simulink model "problem_2c"  (R2018a)
settings: Solver=VariableStepAuto  StartTime=0.0  StopTime=10  MaxStep=1e-3  RelTol=1e-3
values from neighbouring files (symbols this model uses):
  dx0 = 5    [distance_x.m]    (also in grid_search_minimization.m = sqrt(2/m*(Esys-m*g*y0)); minimization.m = sqrt(2/m*(Esys-m*g*y0)); problem_1_script.m; problem_3_script.m = sqrt(2/m*(Esys-m*g*y0)))
  dy0 = 0    [distance_x.m]    (also in grid_search_minimization.m; minimization.m; problem_1_script.m; problem_3_script.m)
  g = 9.81    [distance_x.m]    (also in grid_search_minimization.m; minimization.m; problem_1_script.m; problem_3_script.m)
  ground = 0.00001    (= 1e-05)    [problem_1_script.m]    (also in problem_3_script.m; smm_params.m)
  k = 20000    [distance_x.m]    (also in grid_search_minimization.m = kVec(kIdx); minimization.m; problem_1_script.m = kVec(kIdx); problem_3_script.m)
  l0 = 1    [distance_x.m]    (also in grid_search_minimization.m; minimization.m; problem_1_script.m; problem_3_script.m)
  m = 80    [distance_x.m]    (also in grid_search_minimization.m; minimization.m; problem_1_script.m; problem_3_script.m)
  x0 = 0    [distance_x.m]    (also in grid_search_minimization.m; minimization.m; problem_1_script.m; problem_3_script.m)
  y0 = 1    [distance_x.m]    (also in grid_search_minimization.m = y0Vec(yIdx); minimization.m = y0Vec(yIdx); problem_1_script.m; problem_3_script.m = y0Vec3(yIdx))
undefined symbols (not defined in the file or in its folder): angle_noise
libraries: simulink_extras x1
settings Model: Creator=hgeyer  LastModifiedBy=oliver

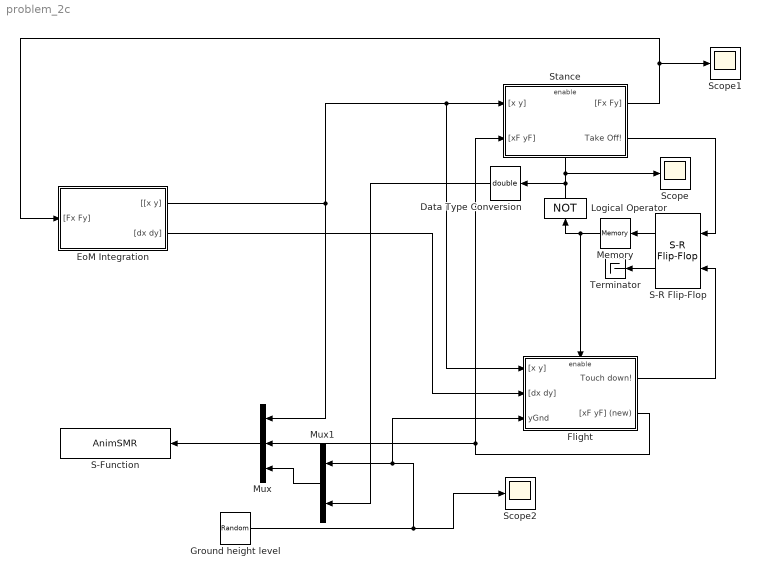
== system problem_2c ==
  " Stance" : Subsystem
  Data Type Conversion : DataTypeConversion  OutDataTypeStr=double
  EoM Integration : Subsystem
  Flight : Subsystem
  Ground height level : UniformRandomNumber  Minimum=-ground  Maximum=ground  SampleTime=0.3
  Logical Operator : Logic  Operator=NOT  AllPortsSameDT=off  OutDataTypeStr=boolean
  Memory : Memory  InitialCondition=1
  Mux : Mux  Inputs=3
  Mux1 : Mux  Inputs=2
  S-Function : S-Function  FunctionName=AnimSMR  Parameters=0.5  SFunctionDeploymentMode=off  EnableBusSupport=off
  S-R Flip-Flop : simulink_extras/Flip Flops/S-R Flip-Flop  initial_condition=1
  Scope : Scope
  Scope1 : Scope
  Scope2 : Scope
  Terminator : Terminator
  wires:
  EoM Integration/1("[[x y]") -> Flight/1("[x y]"), " Stance"/1("[x y]"), Mux/1
  EoM Integration/2("[dx dy]") -> Flight/2("[dx dy]")
  " Stance"/2(Take Off!) -> S-R Flip-Flop/1
  S-R Flip-Flop/1 -> Memory/1
  Logical Operator/1 -> Data Type Conversion/1, " Stance"/Enable, Scope/1
  Memory/1 -> Logical Operator/1, Flight/Enable
  S-R Flip-Flop/2 -> Terminator/1
  Flight/1(Touch down!) -> S-R Flip-Flop/2
  " Stance"/1("[Fx Fy]") -> EoM Integration/1("[Fx Fy]"), Scope1/1
  Flight/2("[xF yF] (new)") -> " Stance"/2("[xF yF]"), Mux/2
  Mux/1 -> S-Function/1
  Mux1/1 -> Mux/3
  Data Type Conversion/1 -> Mux1/2
  Ground height level/1 -> Flight/3(yGnd), Mux1/1, Scope2/1

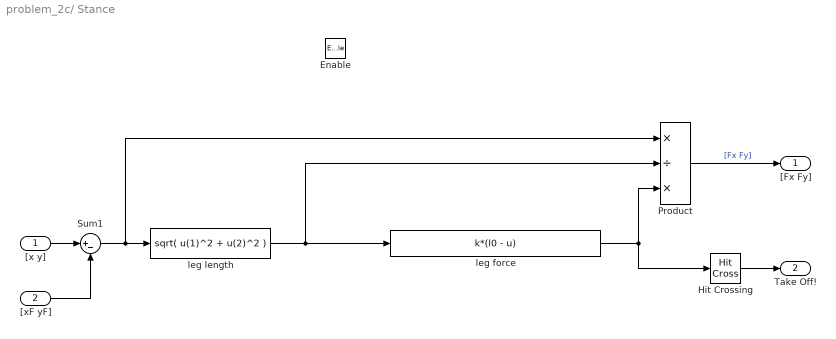
== system problem_2c/ Stance ==
  "[x y]" : Inport
  "[xF yF]" : Inport  Port=2
  Enable : EnablePort
  Hit Crossing : HitCross  HitCrossingDirection=falling
  Product : Product  Inputs=*/*
  Sum1 : Sum  Inputs=|+-
  leg force : Fcn  Expr=k*(l0 - u)
  leg length : Fcn  Expr=sqrt( u(1)^2 + u(2)^2 )
  "[Fx Fy]" : Outport  OutputWhenDisabled=reset  InitialOutput=[0,0]
  Take Off! : Outport  Port=2  OutputWhenDisabled=reset  InitialOutput=0
  wires:
  Product/1 -> "[Fx Fy]"/1  "[Fx Fy]"
  leg length/1 -> leg force/1, Product/2
  Hit Crossing/1 -> Take Off!/1
  "[x y]"/1 -> Sum1/1
  "[xF yF]"/1 -> Sum1/2
  Sum1/1 -> Product/1, leg length/1
  leg force/1 -> Hit Crossing/1, Product/3

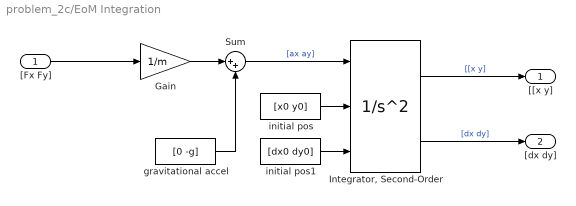
== system problem_2c/EoM Integration ==
  "[Fx Fy]" : Inport
  Gain : Gain  Gain=1/m
  "Integrator, Second-Order" : SecondOrderIntegrator  ICSourceX=external  ICSourceDXDT=external
  Sum : Sum  Inputs=|++
  gravitational accel : Constant  Value=[0 -g]
  initial pos : Constant  Value=[x0 y0]
  initial pos1 : Constant  Value=[dx0 dy0]
  "[[x y]" : Outport
  "[dx dy]" : Outport  Port=2
  wires:
  "[Fx Fy]"/1 -> Gain/1
  initial pos1/1 -> "Integrator, Second-Order"/3
  "Integrator, Second-Order"/2 -> "[dx dy]"/1  "[dx dy]"
  Gain/1 -> Sum/1
  initial pos/1 -> "Integrator, Second-Order"/2
  "Integrator, Second-Order"/1 -> "[[x y]"/1  "[[x y]"
  Sum/1 -> "Integrator, Second-Order"/1  "[ax ay]"
  gravitational accel/1 -> Sum/2

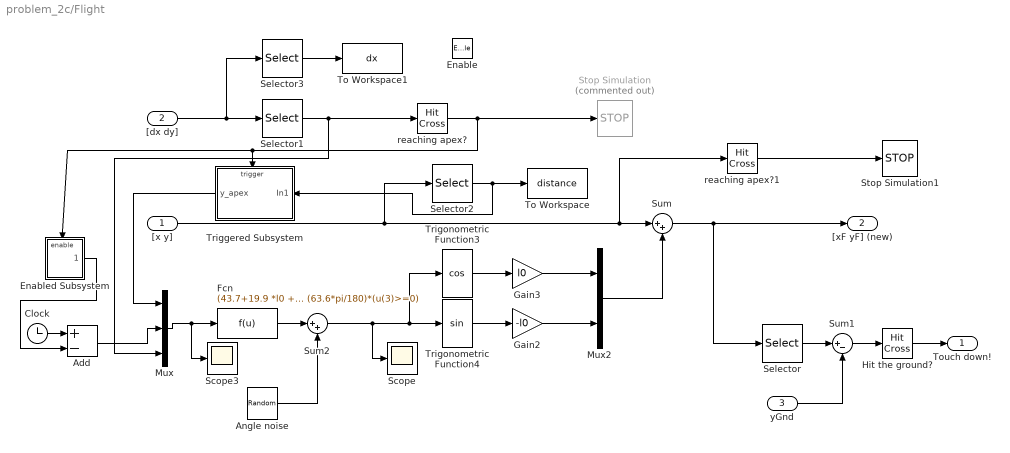
== system problem_2c/Flight ==
  "[x y]" : Inport
  "[dx dy]" : Inport  Port=2
  yGnd : Inport  Port=3
  Enable : EnablePort
  Add : Sum  Inputs=+-
  Angle noise : UniformRandomNumber  Minimum=-angle_noise  Maximum=angle_noise  SampleTime=0.3
  Clock : Clock
  Enabled Subsystem : Subsystem  TreatAsAtomicUnit=on
  Fcn : Fcn  Expr=(43.7+19.9 *l0 + 10.8*g*u(2)^2)*(pi/180)*(u(3)<0) + (63.6*pi/180)*(u(3)>=0)
  Gain2 : Gain  Gain=-l0
  Gain3 : Gain  Gain=l0
  Hit the ground? : HitCross  HitCrossingDirection=falling
  Mux : Mux  Inputs=3
  Mux2 : Mux  Inputs=2
  Scope : Scope
  Scope3 : Scope
  Selector : Selector  InputPortWidth=2  IndexOptions=Index vector (dialog)  Indices=2  OutputSizes=1
  Selector1 : Selector  InputPortWidth=2  IndexOptions=Index vector (dialog)  Indices=2  OutputSizes=1
  Selector2 : Selector  InputPortWidth=2  IndexOptions=Index vector (dialog)  Indices=1  OutputSizes=1
  Selector3 : Selector  InputPortWidth=2  IndexOptions=Index vector (dialog)  Indices=1  OutputSizes=1
  Stop Simulation : Stop  Commented=on
  Stop Simulation1 : Stop
  Sum : Sum  Inputs=|++
  Sum1 : Sum  Inputs=|+-
  Sum2 : Sum  Inputs=|++
  To Workspace : ToWorkspace  VariableName=distance  SampleTime=-1
      settings: MaxDataPoints=1
  To Workspace1 : ToWorkspace  VariableName=dx  SampleTime=-1
  Triggered Subsystem : Subsystem  TreatAsAtomicUnit=on
  Trigonometric Function3 : Trigonometry  Operator=cos
  Trigonometric Function4 : Trigonometry
  reaching apex? : HitCross  HitCrossingOffset=eps  HitCrossingDirection=falling
  reaching apex?1 : HitCross  HitCrossingDirection=falling
  Touch down! : Outport  OutputWhenDisabled=reset  InitialOutput=0
  "[xF yF] (new)" : Outport  Port=2
  wires:
  Trigonometric Function4/1 -> Gain2/1
  Trigonometric Function3/1 -> Gain3/1
  Gain2/1 -> Mux2/2
  Gain3/1 -> Mux2/1
  Mux2/1 -> Sum/2
  "[x y]"/1 -> Selector2/1, reaching apex?1/1, Sum/1
  Sum/1 -> Selector/1, "[xF yF] (new)"/1
  Hit the ground?/1 -> Touch down!/1
  "[dx dy]"/1 -> Selector3/1, Selector1/1
  Selector1/1 -> Mux/3, reaching apex?/1
  reaching apex?/1 -> Enabled Subsystem/Enable, Triggered Subsystem/Trigger, Stop Simulation/1
  Selector2/1 -> Triggered Subsystem/1(In1), To Workspace/1
  Selector3/1 -> To Workspace1/1
  Selector/1 -> Sum1/1
  Sum1/1 -> Hit the ground?/1
  yGnd/1 -> Sum1/2
  Triggered Subsystem/1(y_apex) -> Mux/1
  Mux/1 -> Scope3/1, Fcn/1
  Clock/1 -> Add/1
  Add/1 -> Mux/2
  Enabled Subsystem/1(t_apex) -> Add/2
  reaching apex?1/1 -> Stop Simulation1/1
  Fcn/1 -> Sum2/1
  Sum2/1 -> Scope/1, Trigonometric Function3/1, Trigonometric Function4/1
  Angle noise/1 -> Sum2/2

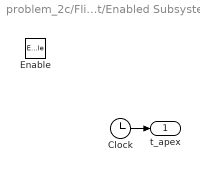
== system problem_2c/Flight/Enabled Subsystem ==
  Enable : EnablePort
  Clock : Clock
  t_apex : Outport
  wires:
  Clock/1 -> t_apex/1

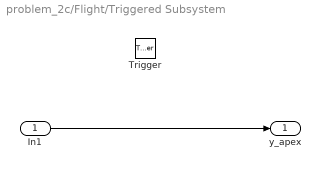
== system problem_2c/Flight/Triggered Subsystem ==
  In1 : Inport
  Trigger : TriggerPort  TriggerType=falling  VariantControl=Variant
  y_apex : Outport
  wires:
  In1/1 -> y_apex/1
